simulink model "disturbance_attenuation_with_observer"  (R2020a)
settings: Solver=VariableStepAuto  StartTime=0.0  StopTime=10  RelTol=1e-10  AbsTol=1e-8
InitFcn:
  | A=[0 1;0 0];
  | B=[0;1];
  | D=1;
  | phi=.7;
  | x0=[2;3];
  | K=place(A,B,[-2 -3]);
  | Aep=[0 1 0 0;0 0 1 0;0 0 0 1;0 0 -1 0];
  | Bep=[0;1;0;0];Cep=[1 0 0 0;0 1 0 0];
  | M=place(Aep',Cep',[-5 -6 -7 -8]);
  | L=M';
  | Ad=3;Bd=-2;wd=3;
settings Model: Creator=Haris  LastModifiedBy=Haris

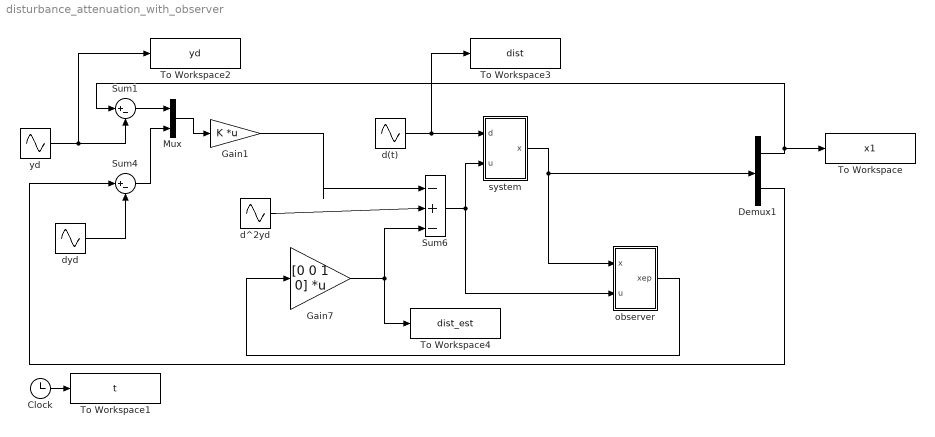
== system disturbance_attenuation_with_observer ==
  Clock : Clock
  Demux1 : Demux  Outputs=2
  Gain1 : Gain  Gain=K  Multiplication=Matrix(K*u)
  Gain7 : Gain  Gain=[0 0 1 0]  Multiplication=Matrix(K*u)
  Mux : Mux  Inputs=2
  Sum1 : Sum  Inputs=|+-
  Sum4 : Sum  Inputs=|+-
  Sum6 : Sum  Inputs=|-+-
  To Workspace : ToWorkspace  VariableName=x1  SampleTime=-1
  To Workspace1 : ToWorkspace  VariableName=t  SampleTime=-1
  To Workspace2 : ToWorkspace  VariableName=yd  SampleTime=-1
  To Workspace3 : ToWorkspace  VariableName=dist  SampleTime=-1
  To Workspace4 : ToWorkspace  VariableName=dist_est  SampleTime=-1
  d(t) : Sin  Amplitude=D  Phase=phi  SampleTime=0
  d^2yd : Sin  Amplitude=Ad*wd^2  Frequency=wd  Phase=pi  SampleTime=0
  dyd : Sin  Amplitude=Ad*wd  Frequency=wd  Phase=pi/2  SampleTime=0
  observer : Subsystem
  system : Subsystem
  yd : Sin  Amplitude=Ad  Bias=Bd  Frequency=wd  SampleTime=0
  wires:
  Demux1/1 -> To Workspace/1, Sum1/1
  Demux1/2 -> Sum4/1
  Clock/1 -> To Workspace1/1
  d(t)/1 -> To Workspace3/1, system/1(d)
  system/1(x) -> observer/1(x), Demux1/1
  yd/1 -> Sum1/2, To Workspace2/1
  dyd/1 -> Sum4/2
  Sum1/1 -> Mux/1
  Sum4/1 -> Mux/2
  Mux/1 -> Gain1/1
  Sum6/1 -> system/2(u), observer/2(u)
  Gain1/1 -> Sum6/1
  d^2yd/1 -> Sum6/2
  Gain7/1 -> To Workspace4/1, Sum6/3
  observer/1(xep) -> Gain7/1

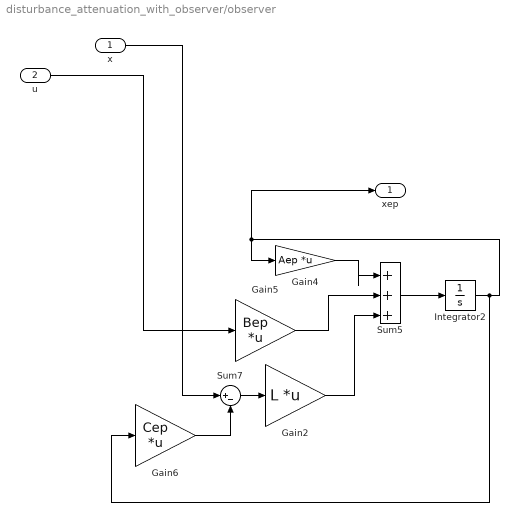
== system disturbance_attenuation_with_observer/observer ==
  x : Inport
  u : Inport  Port=2
  Gain2 : Gain  Gain=L  Multiplication=Matrix(K*u)
  Gain4 : Gain  Gain=Aep  Multiplication=Matrix(K*u)
  Gain5 : Gain  Gain=Bep  Multiplication=Matrix(K*u)
  Gain6 : Gain  Gain=Cep  Multiplication=Matrix(K*u)
  Integrator2 : Integrator  InitialCondition=[0;0;0;0]
  Sum5 : Sum  Inputs=|+++
  Sum7 : Sum  Inputs=|+-
  xep : Outport
  wires:
  Gain6/1 -> Sum7/2
  Integrator2/1 -> Gain6/1, xep/1, Gain4/1
  x/1 -> Sum7/1
  Gain4/1 -> Sum5/1
  Gain5/1 -> Sum5/2
  Gain2/1 -> Sum5/3
  Sum7/1 -> Gain2/1
  u/1 -> Gain5/1
  Sum5/1 -> Integrator2/1

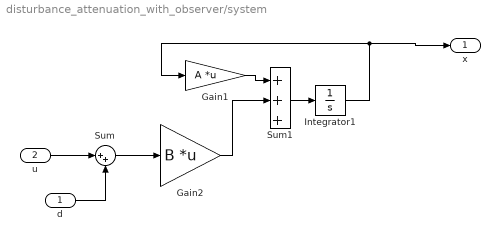
== system disturbance_attenuation_with_observer/system ==
  d : Inport
  u : Inport  Port=2
  Gain1 : Gain  Gain=A  Multiplication=Matrix(K*u)
  Gain2 : Gain  Gain=B  Multiplication=Matrix(K*u)
  Integrator1 : Integrator  InitialCondition=x0
  Sum : Sum  Inputs=|++
  Sum1 : Sum  Inputs=|+++
  x : Outport
  wires:
  Integrator1/1 -> Gain1/1, x/1
  Gain1/1 -> Sum1/1
  Sum1/1 -> Integrator1/1
  Gain2/1 -> Sum1/2
  u/1 -> Sum/1
  Sum/1 -> Gain2/1
  d/1 -> Sum/2
